simulink model "step4-d"  (R2020b)
settings: Solver=VariableStepAuto  StartTime=0.0  StopTime=10.0  RelTol=1e-3
libraries: dspadpt3 x1, dspsrcs4 x1
settings Model: Creator=Borma  LastModifiedBy=Borma

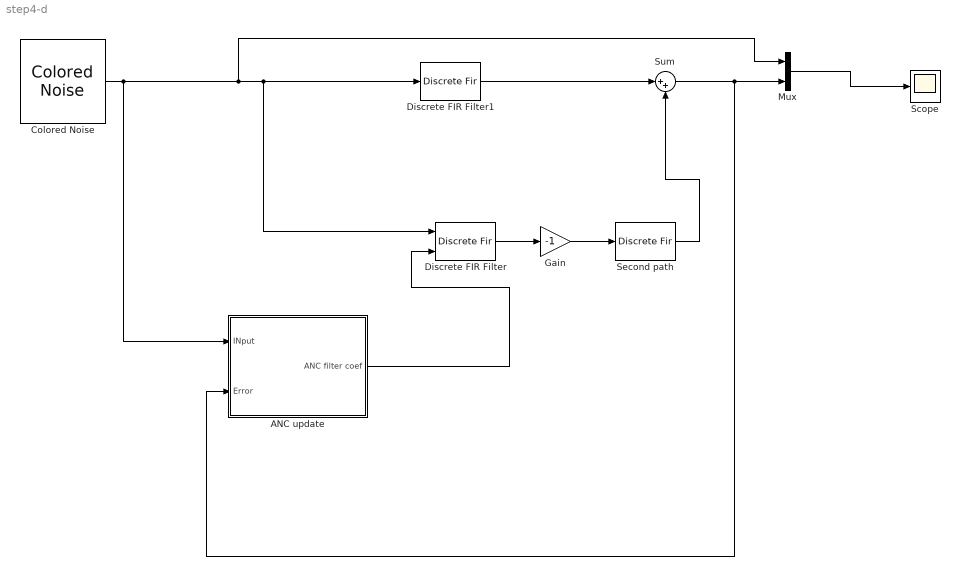
== system step4-d ==
  ANC update : Subsystem
  Colored Noise : dspsrcs4/Colored Noise  Color=white  InverseFrequencyPower=1  BoundedOutput=on  NumChannels=1  OutputDataType=double  SamplesPerFrame=1  SampleTime=1/4000  RandomStream=mt19937ar with seed  Seed=67  SimulateUsing=Interpreted execution
      settings: SourceProductBaseCode=DS
  Discrete FIR Filter : DiscreteFir  CoefSource=Input port  InputProcessing=Columns as channels (frame based)
      settings: InputPortMap=u0,u1
  Discrete FIR Filter1 : DiscreteFir  Coefficients=[0.5 0.1 0.2 0.4 0 0 -0.125 0.3 0.5 0 0.075 -0.25 -0.4]
  Gain : Gain  Gain=-1
  Mux : Mux  Inputs=2
  Scope : Scope
  Second path : DiscreteFir  Coefficients=[0 0 -0.5 -0.5 -0.3 0.2 -0.1 0.5 -0.5]
  Sum : Sum  Inputs=|++
  wires:
  Colored Noise/1 -> ANC update/1(INput), Mux/1, Discrete FIR Filter/1, Discrete FIR Filter1/1
  Second path/1 -> Sum/2
  Discrete FIR Filter1/1 -> Sum/1
  Gain/1 -> Second path/1
  Sum/1 -> ANC update/2(Error), Mux/2
  Discrete FIR Filter/1 -> Gain/1
  ANC update/1(ANC filter coef) -> Discrete FIR Filter/2
  Mux/1 -> Scope/1

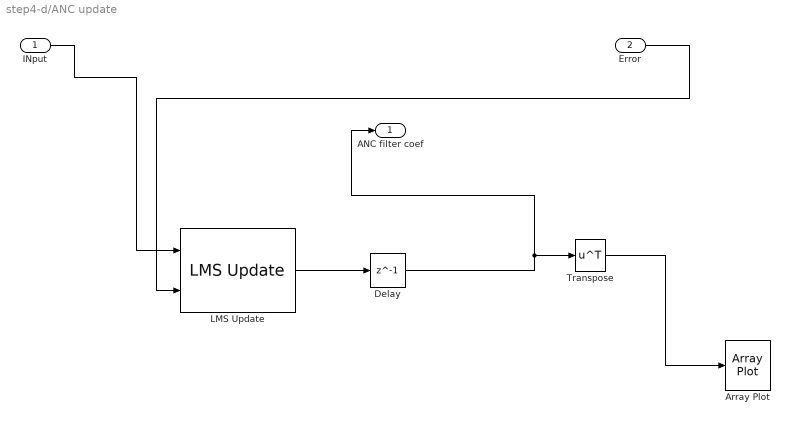
== system step4-d/ANC update ==
  INput : Inport
  Error : Inport  Port=2
  Array Plot : ArrayPlot
  Delay : Delay  DelayLength=1  InitialCondition=0
  LMS Update : dspadpt3/LMS Update  Method=Normalized LMS  Length=24  StepSizeSource=Property  StepSize=0.01  LeakageFactor=1.0  InitialConditions=0  EnableAdaptInput=off  EnableResetInput=off  SimulateUsing=Code generation
      settings: SourceProductBaseCode=DS
  Transpose : Math  Operator=transpose  SaturateOnIntegerOverflow=on
  ANC filter coef : Outport
  wires:
  INput/1 -> LMS Update/1
  Delay/1 -> ANC filter coef/1, Transpose/1
  Transpose/1 -> Array Plot/1
  LMS Update/1 -> Delay/1
  Error/1 -> LMS Update/2
